simulink model "copy"  (R2021a)
settings: Solver=VariableStepAuto  StartTime=0.0  StopTime=inf  FixedStep=1  RelTol=1e-3
undefined symbols (not defined in the file or in its folder): f, gray
libraries: instrumentlib x3, pid_lib x1
settings Model: SnapshotBufferSize=1000000  Creator=花舞  LastModifiedBy=LYC
settings SolverCC: AlgebraicLoopSolver=TrustRegion
settings OptimizationCC: OptimizeBlockIOStorage=off  OptimizeDataStoreBuffers=off  BusAssignmentInplaceUpdate=off
settings DebuggingCC: SFUnexpectedBacktrackingDiag=warning  SFNoUnconditionalDefaultTransitionDiag=warning  SFMachineParentedDataDiag=warning
settings RTWCC: GenerateReport=on  BuildConfiguration=Debug  LaunchReport=on
settings CodeAppCC: ForceParamTrailComments=on  MATLABSourceComments=on  EnableCustomComments=on
settings GRTTargetCC: CombineSignalStateStructs=on  SupportVariableSizeSignals=on  MultiInstanceErrorCode=Warning

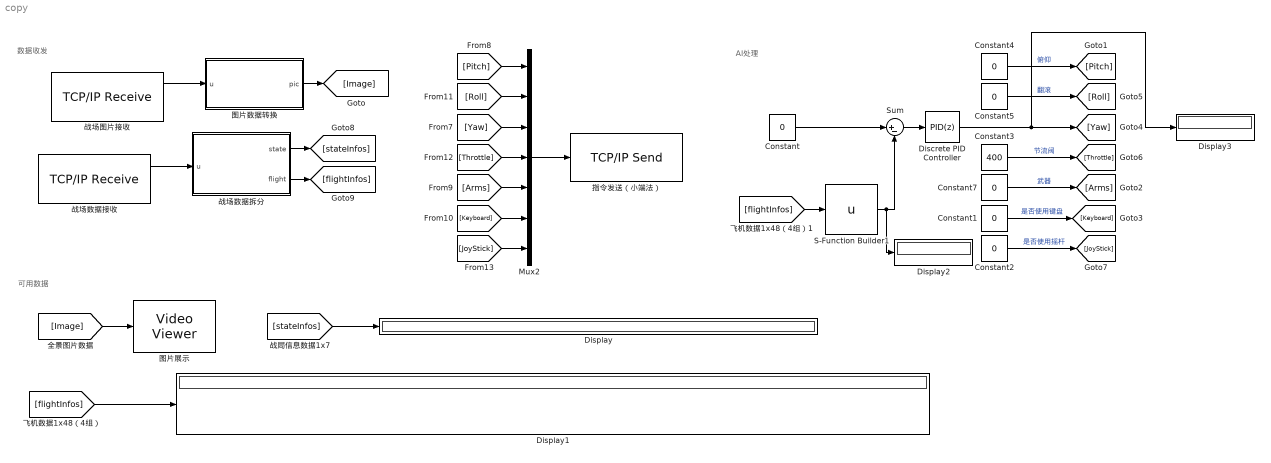
== system copy ==
  note: AI处理
  note: 可用数据
  note: 数据收发
  Constant : Constant  Value=0  OutDataTypeStr=double
  Constant{1..2,4..5,7} (5 alike) : Constant  Value=0  OutDataTypeStr=int32
  Constant3 : Constant  Value=400  OutDataTypeStr=int32
  Discrete PID Controller : pid_lib/PID Controller  Controller=PID  Form=Parallel  TimeDomain=Discrete-time  UseExternalTs=off  SampleTime=-1  IntegratorMethod=Forward Euler  FilterMethod=Forward Euler  ControllerParametersSource=internal  P=100  I=0  D=0  UseFilter=on  N=100  TunerSelectOption=Transfer Function Based (PID Tuner App)  InitialConditionSource=internal  InitialConditionForIntegrator=0  InitialConditionForFilter=0  DifferentiatorICPrevScaledInput=0  ExternalReset=none  TrackingMode=off  Kt=1  LimitOutput=on  SatLimitsSource=internal  UpperSaturationLimit=1000  LowerSaturationLimit=-1000  LinearizeAsGain=off  AntiWindupMode=none  Kb=1  RndMeth=Ceiling  POutMin=[]  POutMax=[]  IOutMin=[]  IOutMax=[]  DOutMin=[]  DOutMax=[]  NOutMin=[]  NOutMax=[]  SumOutDataTypeStr=int32  SumOutMin=[]  SumOutMax=[]  SaturationOutMin=[]  SaturationOutMax=[]  PParamMin=[]  PParamMax=[]  IParamMin=[]  IParamMax=[]  DParamMin=[]  DParamMax=[]  NParamMin=[]  NParamMax=[]  KbParamMin=[]  KbParamMax=[]  KtParamMin=[]  KtParamMax=[]  KbOutMin=[]  KbOutMax=[]  KtOutMin=[]  KtOutMax=[]  IntegratorOutMin=[]  IntegratorOutMax=[]  FilterOutMin=[]  FilterOutMax=[]  SumI1OutMin=[]  SumI1OutMax=[]  SumI2OutMin=[]  SumI2OutMax=[]  SumI3OutMin=[]  SumI3OutMax=[]  SumI4OutMin=[]  SumI4OutMax=[]  SumDOutMin=[]  SumDOutMax=[]  DifferentiatorOutMin=[]  DifferentiatorOutMax=[]  FilterDiffOutCoefMin=[]  FilterDiffOutCoefMax=[]  ReciprocalOutMin=[]  ReciprocalOutMax=[]  SumDenOutMin=[]  SumDenOutMax=[]  SumNumOutMin=[]  SumNumOutMax=[]  DivideOutMin=[]  DivideOutMax=[]  UdiffTsProdOutMin=[]  UdiffTsProdOutMax=[]  NTsProdOutMin=[]  NTsProdOutMax=[]  UintegralTsProdOutMin=[]  UintegralTsProdOutMax=[]  UngainTsProdOutMin=[]  UngainTsProdOutMax=[]  IntegratorContinuousStateAttributes=''  IntegratorStateMustResolveToSignalObject=off  IntegratorRTWStateStorageClass=Auto  FilterContinuousStateAttributes=''  FilterStateMustResolveToSignalObject=off  FilterRTWStateStorageClass=Auto  ParallelPVariant=InternalParameters  IdealPVariant=Disabled  IVariant=InternalParameters  DVariant=InternalParameters  IntegratorVariant=Discrete  SatVariant=Enabled  AWVariant=Passthrough  PCopyVariant=Disabled  TRVariant=Disabled  FdbkBlocksVariant=Forward  IdealPFdbkVariant=Disabled  SatFdbkVariant=Disabled  DerivativeFilterVariant=ForwardEulerFilter  NVariant=InternalParameters  NCopyVariant=Disabled  FilterICVariant=InternalICsFilter  IntegratorICVariant=InternalICs  ExternalResetVariant=Disabled  TRSumVariant=Passthrough  SumFdbkVariant=Disabled  SumVariant=Sum_PID  TsampFilterVariant=InternalTs  TsampNgainVariant=Passthrough  TsampIntegralVariant=Passthrough  ExternalSaturationOutDataTypeStr=Inherit: Same as second input
  Display{,1..3} (4 alike) : Display
  Mux2 : Mux  Inputs=7
  S-Function Builder1 : S-Function  FunctionName=u  SFunctionModules=u_wrapper  SFunctionDeploymentMode=off  EnableBusSupport=off  mask(S-Function Builder){}
      mask help: Simulink:masks:SFunctionBuilder_MD
      mask init:
      | val = [[.9  0.75 0.75 1 1 .9 .9 1]',[1 1 0.75 0.75 .9 .9 1 .9]'];try , sys = get_param(gcb,'SfunBuilderFcnName');if isempty(sys), sys = get_param(gcb,'FunctionName'); end,catch, sys = get_param(gcb,'FunctionName'); end
      settings: CopyFcn=set_param(gcbh,'LinkStatus','none')  OpenFcn=sfunctionwizard(gcbh)
      mask Display:
      | plot(val(:,1),val(:,2))
      | disp(sys)
      | port_label('input',1,'u0')
      | port_label('output',1,'y0')
  Sum : Sum  Inputs=|+-
  图片展示 : VideoViewer  colormapValue=gray(256)  FigPos=[-59 756 1282.66666666667 624.666666666667]
  图片数据转换 : MATLAB Function  TreatAsAtomicUnit=on
  战场图片接收 : instrumentlib/TCP//IP Receive  Host=0.0.0.0  Port=9999  DataSize="[1  1572864]"  EnableBlockingMode=off  Timeout=10  SampleTime=0.01  DataType=uint8  ByteOrder=BigEndian  ASCIIFormatting=%f,  Terminator=LF
  战场数据拆分 : MATLAB Function  TreatAsAtomicUnit=on
  战场数据接收 : instrumentlib/TCP//IP Receive  Host=0.0.0.0  Port=10000  DataSize="[1  55]"  EnableBlockingMode=off  Timeout=10  SampleTime=0.01  DataType=int32  ByteOrder=LittleEndian  ASCIIFormatting=%f,  Terminator=LF
  指令发送（小端法） : instrumentlib/TCP//IP Send  Host=0.0.0.0  Port=9999  EnableBlockingMode=off  Timeout=10  ByteOrder=LittleEndian  TransferDelay=on
  wires:
  Constant4/1 -> [Pitch]  "俯仰"
  Constant5/1 -> [Roll]  "翻滚"
  Constant3/1 -> [Throttle]  "节流阀"
  Constant7/1 -> [Arms]  "武器"
  Constant1/1 -> [Keyboard]  "是否使用键盘"
  Constant2/1 -> [JoyStick]  "是否使用摇杆"
  [Keyboard] -> Mux2/6
  [Roll] -> Mux2/2
  [Pitch] -> Mux2/1
  [Throttle] -> Mux2/4
  [Yaw] -> Mux2/3
  [Arms] -> Mux2/5
  [JoyStick] -> Mux2/7
  Mux2/1 -> 指令发送（小端法）/1
  [stateInfos] -> Display/1
  [flightInfos] -> Display1/1
  战场数据接收/1 -> 战场数据拆分/1(u)
  战场数据拆分/1(state) -> [stateInfos]
  战场数据拆分/2(flight) -> [flightInfos]
  [flightInfos] -> S-Function Builder1/1
  Constant/1 -> Sum/1
  Discrete PID Controller/1 -> Display3/1, [Yaw]
  Sum/1 -> Discrete PID Controller/1
  S-Function Builder1/1 -> Display2/1, Sum/2
  图片数据转换/1(pic) -> [Image]
  战场图片接收/1 -> 图片数据转换/1(u)
  [Image] -> 图片展示/1

== matlab function copy/战场数据拆分 ==
  data: u input; state output; flight output
function [state,flight] = fcn(u)
state = u(1:7);
flight = u(8:end);

== matlab function copy/图片数据转换 ==
  data: u input; pic output
function pic = fcn(u)
coder.extrinsic('image');
col = 1024;
row = 512;
temp = 1;
I = zeros(row, col, 3);
for i=1:row
    for j=1:col
        I(513 - i,j,1)=u(temp);
        I(513 - i,j,2)=u(temp+1);
        I(513 - i,j,3)=u(temp+2);
        temp = temp + 3;
    end
end
pic = double(I)/255;
